simulink model "Aplicacion"  (Simulink 9.1)
settings: Solver=ode45  StartTime=0.0  StopTime=30  RelTol=1e-3  AbsTol=1e-6
values from neighbouring files (symbols this model uses):
  b0 = 3    [sys.m]
  b1 = 3    [sys.m]
  b2 = 4    [sys.m]
  b3 = 2    [sys.m]
  k = 3    [sys.m]
undefined symbols (not defined in the file or in its folder): sfunxy2
libraries: neural x1
settings Model: SuppressorTable=22 serialization::archive 11 0 6 0 0 0 1 0  Creator=munlock -all d:\work\myr12\toolbox\fuzzy\fuzzy\mfedit.m  LastModifiedBy=daniel  ExtModeTrigMode=oneshot  ExtModeArmWhenConnect=off  TunableVars=prueba  TunableVarsStorageClass=Auto
settings SolverCC: AutoScaleAbsTol=off
settings DataIOCC: SignalLoggingSaveFormat=ModelDataLogs  SaveOutput=off  SignalLoggingName=sigsOut
settings OptimizationCC: BooleanDataType=off  InitFltsAndDblsToZero=on
settings DebuggingCC: SaveWithParameterizedLinksMsg=none  SignalResolutionControl=TryResolveAllWithWarning  MultiTaskDSMMsg=warning  MultiTaskCondExecSysMsg=none
settings HardwareCC: TargetUnknown=on
settings RTWCC: TemplateMakefile=grt_vc.tmf
settings GRTTargetCC: TargetFcnLib=ansi_tfl_tmw.mat

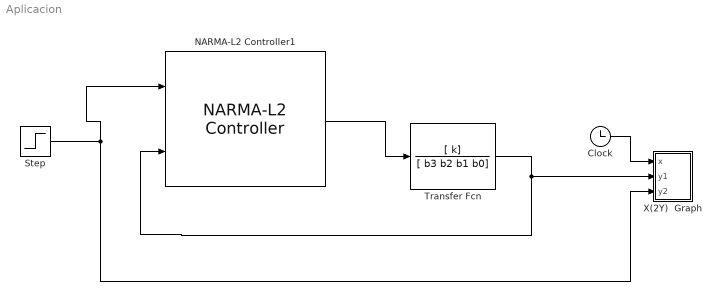
== system Aplicacion ==
  Clock : Clock
  NARMA-L2 Controller1 : neural/Control Systems/NARMA-L2 Controller  Normalize=1  IW1_1=[-1.2113105830470793922 -0.38286971145025922025 -0.03593760462771073555 -1.2948000628602196471 -1.9087199868979829454;-1.0240065522962886746 -0.89290276831461656837 0.57609152819189135553 -0.06962432489502770605 -0.2794966310487509431;0.36275463922878142808 1.4277190141768851817 -0.77146090067182471195 -0.054097038026323138182 -0.9568090642166328097;-0.44221525728340860262 1.3022121711888940965 1.2174275071589253372 -0.15267159784880413032 -0.70000003129219312559]  IW3_2=[-0.54684099020283971626 -1.2326776123507758864 -0.18274174231776454946 -1.1583859422614253276 0.4677173718071272468;1.2086132618397449345 0.56109212474900471701 0.17688443538235873453 0.70279805301792042105 1.0544393288578464141;-1.150339229428901433 0.55004403127043410837 -0.48349455072011765511 -0.75130383270801115447 -0.99432149032556371715;-1.203297284871107653 0.389031593725764957 0.64430213462204621866 -0.34629222790387576003 1.1306247050677740162]  IW5_3=0.015068068678347210435  LW2_1=[0.91331574829390294035 0.94357236418457979266 -1.563398601900424234 -0.10767300675880130123]  LW4_3=[0.55120811407070913202 -0.02648542352943836567 -0.12814737720229038564 -0.10657942756163264753]  LW5_4=0.014863913740404660624  LW6_5=0.58935776694487518323  LW6_2=-0.55142028923153274533  B1=[1.1470095899987249322;-0.11488869862095513197;0.067028113693047591815;-2.6975372525937006962]  B2=0.0040217688256677167069  B3=[1.8472801390176727399;-0.6157975376300928172;-0.6157258596481404167;-1.8472878399866565768]  B4=-0.38714579917001434861  Limit_output=0  min_output=-Inf  max_output=Inf  Use_Previous_Weights=1  Ts=0.03  S1=4  Ni=3  Nj=3  sim_file=ModeloPlanta  trainfun=trainlm  Use_validation=1  Use_Testing=1  max_i=10  min_i=0  max_i_int=10  min_i_int=1  sam_training=800  epochs=1200  minp=1.6218230819324275238  maxp=3.1121504204480485711  mint=0  maxt=3.1121504204480485711
      settings: SourceProductName=Neural Network Toolbox  SourceProductBaseCode=NN
  Step : Step  Time=0  SampleTime=0
  Transfer Fcn : TransferFcn  Numerator=[ k]  Denominator=[ b3 b2 b1 b0]
  X(2Y)  Graph : Subsystem  LoadFcn=sfunxy2([],[],[],'LoadBlock')  StartFcn=sfunxy2([],[],[],'Start')  StopFcn=sfunxy2([],[],[],'Stop')  mask(X(2Y) scope.){xmin=0, xmax=10, ymin=0, ymax=2, st=-1}
      mask prompts: xmin "x-min:"; xmax "x-max:"; ymin "y-min:"; ymax "y-max:"; st "Sample time:"
      mask help: X(2Y) scope using MATLAB graph window. First input is used as time base. Enter plotting ranges.
      settings: CopyFcn=sfunxy2([],[],[],'CopyBlock')  DeleteFcn=sfunxy2([],[],[],'DeleteBlock')  NameChangeFcn=sfunxy2([],[],[],'NameChange')
      mask Help: This block can be used to explore limit cycles. Look at the m-file sfunxy.m to see how it works.
      mask Display: plot([.05 .95 .95 .05 .05],[.45 .45 .95 .95 .45], 0.5+cos(0:0.1:2*pi)*0.3,0.7+sin(0:0.1:2*pi)*0.2)
  wires:
  Clock/1 -> X(2Y)  Graph/1(x)
  Step/1 -> NARMA-L2 Controller1/1, X(2Y)  Graph/3(y2)
  Transfer Fcn/1 -> NARMA-L2 Controller1/2, X(2Y)  Graph/2(y1)
  NARMA-L2 Controller1/1 -> Transfer Fcn/1

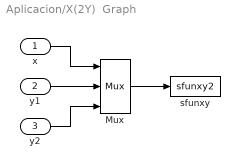
== system Aplicacion/X(2Y)  Graph ==
  x : Inport
  y1 : Inport  Port=2
  y2 : Inport  Port=3
  Mux : Mux  Inputs=3
  sfunxy : S-Function  FunctionName=sfunxy2  Parameters=[xmin xmax ymin ymax], st  SFunctionDeploymentMode=off  EnableBusSupport=off
  wires:
  y2/1 -> Mux/3
  y1/1 -> Mux/2
  x/1 -> Mux/1
  Mux/1 -> sfunxy/1
